simulink model "mode_design"  (R2021a)
settings: Solver=FixedStepDiscrete  StartTime=0.0  StopTime=10.0  FixedStep=0.1  RelTol=1e-3  EnableMultiTasking=on
settings Model: Creator=afonso.miguel  LastModifiedBy=afonso.miguel
settings SolverCC: AlgebraicLoopSolver=TrustRegion  AutoInsertRateTranBlk=on
settings DataIOCC: LimitDataPoints=on
settings OptimizationCC: LifeSpan=inf
settings DebuggingCC: AllowSymbolicDim=off  SFUnexpectedBacktrackingDiag=warning  SFNoUnconditionalDefaultTransitionDiag=warning  SFExecutionAtInitializationDiag=none  ArithmeticOperatorsInVariantConditions=warning
settings SFSimCC: SimUseLocalCustomCode=off  CustomCodeUndefinedFunction=UseInterfaceOnly
settings RTWCC: RTWUseLocalCustomCode=off
settings CodeAppCC: StateflowObjectComments=on
settings GRTTargetCC: TargetLangStandard=C89/C90 (ANSI)
settings ConfigComp: CovMetricSettings=dw  CovSaveCumulativeToWorkspaceVar=on  CovSaveSingleToWorkspaceVar=on  CovExternalEMLEnable=off  CovSFcnEnable=off

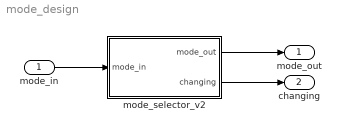
== system mode_design ==
  mode_in : Inport  OutDataTypeStr=fixdt(0,2,0)
  mode_selector_v2 : Stateflow chart  TreatAsAtomicUnit=on
  mode_out : Outport  OutMin=0  OutMax=3  OutDataTypeStr=fixdt(0,2,0)
  changing : Outport  Port=2  OutMin=0  OutMax=1  OutDataTypeStr=fixdt(0,1,0)
  wires:
  mode_in/1 -> mode_selector_v2/1(mode_in)
  mode_selector_v2/1(mode_out) -> mode_out/1
  mode_selector_v2/2(changing) -> changing/1

== stateflow chart mode_design/mode_selector_v2 ==
  settings: executeAtInitialization=1
  state init
  state WaitingChange
  state Step1
    entry:
    mode_buffer1=mode_in;
  state Step2
  (default) -> init
  init -> WaitingChange : {mode_out=0; changing=1;}
  WaitingChange -> WaitingChange [order 1] : [mode_in==mode_out]
      | {changing=0}
  Step2 -> WaitingChange [order 2] : {mode_out=mode_buffer2}
  WaitingChange -> Step1 [order 2] : {changing=1;}
  Step2 -> Step1 [order 1] : [mode_in~=mode_buffer2]
  Step1 -> Step1 [order 1] : [mode_in~=mode_buffer1]
  Step1 -> Step2 [order 2] : {mode_buffer2=mode_in;}
  data: mode_out output fixdt(0,2,0); mode_in input fixdt(0,2,0); mode_buffer1 local fixdt(0,2,0); mode_buffer2 local fixdt(0,2,0); changing output fixdt(0,1,0)
